simulink library "Date"  (R2014b)
settings: Solver=ode45  StartTime=0.0  StopTime=10.0  RelTol=1e-3
undefined symbols (not defined in the file): ConfParam
settings Model: Creator=Hp  LastModifiedBy=Hp

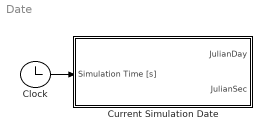
== system Date ==
  Clock : Clock
      settings: Decimation=1/ConfParam.confOrbit.dt
  Current Simulation Date : Subsystem
  wires:
  Clock/1 -> Current Simulation Date/1(Simulation Time [s])

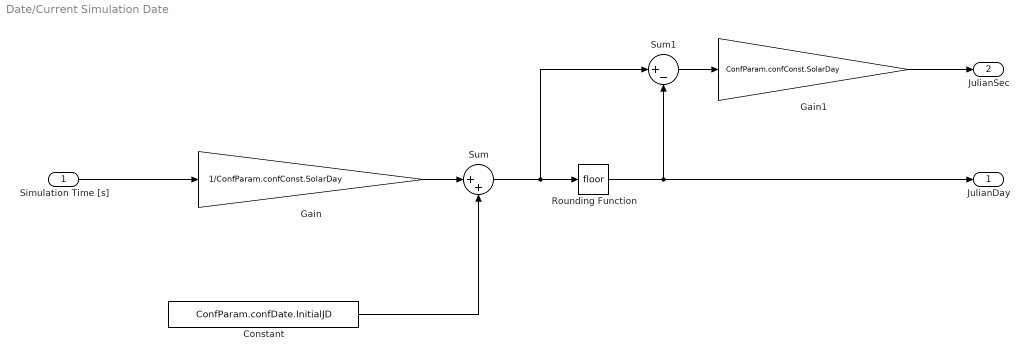
== system Date/Current Simulation Date ==
  Simulation Time [s] : Inport
  Constant : Constant  Value=ConfParam.confDate.InitialJD
  Gain : Gain  Gain=1/ConfParam.confConst.SolarDay
  Gain1 : Gain  Gain=ConfParam.confConst.SolarDay
  Rounding Function : Rounding
  Sum : Sum  Inputs=|++
  Sum1 : Sum  Inputs=|+-
  JulianDay : Outport
  JulianSec : Outport  Port=2
  wires:
  Gain1/1 -> JulianSec/1
  Sum1/1 -> Gain1/1
  Rounding Function/1 -> Sum1/2, JulianDay/1
  Sum/1 -> Rounding Function/1, Sum1/1
  Constant/1 -> Sum/2
  Gain/1 -> Sum/1
  Simulation Time [s]/1 -> Gain/1
